simulink model "RST4"  (R2018a)
settings: Solver=VariableStepAuto  StartTime=0.0  StopTime=50  RelTol=1e-3
values from neighbouring files (symbols this model uses):
  A = den    [cod_teste_RST_4.m]
  B = num    [cod_teste_RST_4.m]
  ep = 0.9    [cod_teste_RST_4.m]
  p3 = Ap3(2)    [cod_teste_RST_4.m]
  p4 = Ap4(2)    [cod_teste_RST_4.m]
  R = [X(5) X(6) X(7) X(8)]    [cod_teste_RST_4.m]
  S = [X(1) X(2) X(3) X(4)]    [cod_teste_RST_4.m]
  T = sum(Am)/sum(B)    [cod_teste_RST_4.m]
  Ta = 0.1    [cod_teste_RST_4.m]
  tc = 1    [cod_teste_RST_4.m]
  Ts = 1    [cod_teste_RST_4.m]
libraries: dspinverses x1
settings Model: Creator=tarci  LastModifiedBy=tarci

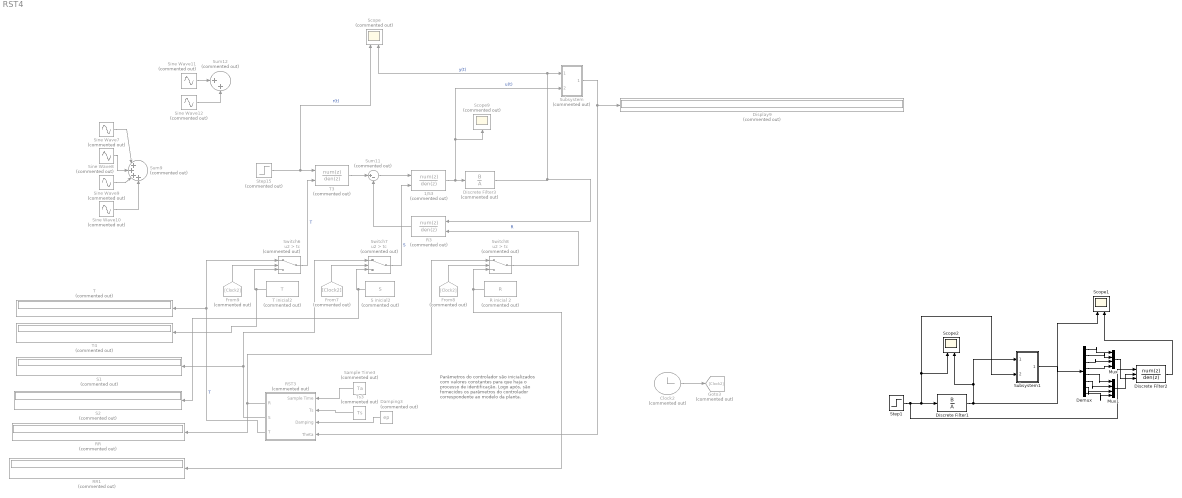
== system RST4 ==
  note: Parâmetros do controlador são inicializados
      | com valores constantes para que haja o
      | processo de identificação. Logo após, são
      | fornecidos os parâmetros do controlador
      | correspondente ao modelo da planta.
  1/S3 : DiscreteFilter  Commented=on  Numerator=1  DenominatorSource=Input port  Denominator=1  a0EqualsOne=on
      settings: InputPortMap=u0,p3
  Clock2 : Clock  Commented=on
  Damping3 : Constant  Commented=on  Value=ep
  Demux : Demux  Outputs=8
  Discrete Filter1 : DiscreteFilter  Numerator=B  Denominator=A  a0EqualsOne=on
  Discrete Filter2 : DiscreteFilter  NumeratorSource=Input port  Numerator=B  DenominatorSource=Input port  Denominator=A  a0EqualsOne=on
      settings: InputPortMap=u0,p1,p3
  Discrete Filter3 : DiscreteFilter  Commented=on  Numerator=B  Denominator=A  a0EqualsOne=on
  Display9 : Display  Commented=on
  From7 : From  Commented=on  GotoTag=Clock2
  From8 : From  Commented=on  GotoTag=Clock2
  From9 : From  Commented=on  GotoTag=Clock2
  Goto3 : Goto  Commented=on  GotoTag=Clock2
  Mux : Mux
  Mux1 : Mux
  R inicial 2 : Constant  Commented=on  Value=R
  R3 : DiscreteFilter  Commented=on  NumeratorSource=Input port  Numerator=[-620.2 131.3]  Denominator=1
      settings: InputPortMap=u0,p1
  RR : Display  Commented=on
  RR1 : Display  Commented=on
  RST3 : Subsystem  Commented=on
  S inicial2 : Constant  Commented=on  Value=S
  S1 : Display  Commented=on
  S2 : Display  Commented=on
  Sample Time3 : Constant  Commented=on  Value=Ta
  Scope : Scope  Commented=on  NumInputPorts=2
  Scope1 : Scope  NumInputPorts=2
  Scope2 : Scope  NumInputPorts=2
  Scope9 : Scope  Commented=on
  Sine Wave10 : Sin  Commented=on  Frequency=8  SampleTime=0
  Sine Wave11 : Sin  Commented=on  SampleTime=0
  Sine Wave12 : Sin  Commented=on  Frequency=2  SampleTime=0
  Sine Wave7 : Sin  Commented=on  SampleTime=0
  Sine Wave8 : Sin  Commented=on  Frequency=2  SampleTime=0
  Sine Wave9 : Sin  Commented=on  Frequency=4  SampleTime=0
  Step1 : Step  Time=0  SampleTime=0
  Step15 : Step  Commented=on  Time=0  SampleTime=0
  Subsystem : Subsystem  Commented=on
  Subsystem1 : Subsystem
  Sum11 : Sum  Commented=on  Inputs=|+-
  Sum12 : Sum  Commented=on  Inputs=|++
  Sum9 : Sum  Commented=on  Inputs=|++++
  Switch6 : Switch  Commented=on  Criteria=u2 > Threshold  Threshold=tc
  Switch7 : Switch  Commented=on  Criteria=u2 > Threshold  Threshold=tc
  Switch8 : Switch  Commented=on  Criteria=u2 > Threshold  Threshold=tc
  T : Display  Commented=on
  T inicial2 : Constant  Commented=on  Value=T
  T3 : DiscreteFilter  Commented=on  NumeratorSource=Input port  Numerator=13.39  Denominator=1
      settings: InputPortMap=u0,p1
  T4 : Display  Commented=on
  Ts3 : Constant  Commented=on  Value=Ts
  wires:
  Step15/1 -> Scope/1, T3/1  "r(t)"
  Sine Wave11/1 -> Sum12/1
  Discrete Filter3/1 -> R3/1, Subsystem/1(y(t)), Scope/2  "y(t)"
  Switch8/1 -> R3/2  "R"
  Sine Wave7/1 -> Sum9/1
  Sine Wave9/1 -> Sum9/3
  From9/1 -> Switch6/2
  Sine Wave8/1 -> Sum9/2
  T inicial2/1 -> T4/1, Switch6/3
  From7/1 -> Switch7/2
  1/S3/1 -> Subsystem/2("u(t) "), Scope9/1, Discrete Filter3/1  "u(t)"
  Subsystem/1("Theta(t) ") -> RST3/4(Theta), Display9/1
  T3/1 -> Sum11/1
  R3/1 -> Sum11/2
  Switch7/1 -> 1/S3/2  "S"
  Clock2/1 -> Goto3/1
  R inicial 2/1 -> RR1/1, Switch8/3
  Sum11/1 -> 1/S3/1
  Sine Wave12/1 -> Sum12/2
  Ts3/1 -> RST3/2(Ts)
  From8/1 -> Switch8/2
  Damping3/1 -> RST3/3(Damping)
  Sample Time3/1 -> RST3/1(Sample Time)
  RST3/3(T) -> Switch6/1, T/1  "T"
  RST3/1(R) -> Switch8/1, RR/1
  Sine Wave10/1 -> Sum9/4
  RST3/2(S) -> Switch7/1, S1/1
  S inicial2/1 -> S2/1, Switch7/3
  Switch6/1 -> T3/2  "T"
  Discrete Filter1/1 -> Scope1/1, Subsystem1/1(y(t)), Scope2/2
  Step1/1 -> Discrete Filter2/1, Subsystem1/2("u(t) "), Scope2/1, Discrete Filter1/1
  Subsystem1/1("Theta(t) ") -> Demux/1
  Demux/1 -> Mux/1
  Demux/2 -> Mux/2
  Demux/3 -> Mux/3
  Demux/4 -> Mux/4
  Demux/5 -> Mux1/1
  Demux/6 -> Mux1/2
  Demux/7 -> Mux1/3
  Demux/8 -> Mux1/4
  Mux1/1 -> Discrete Filter2/2
  Mux/1 -> Discrete Filter2/3
  Discrete Filter2/1 -> Scope1/2

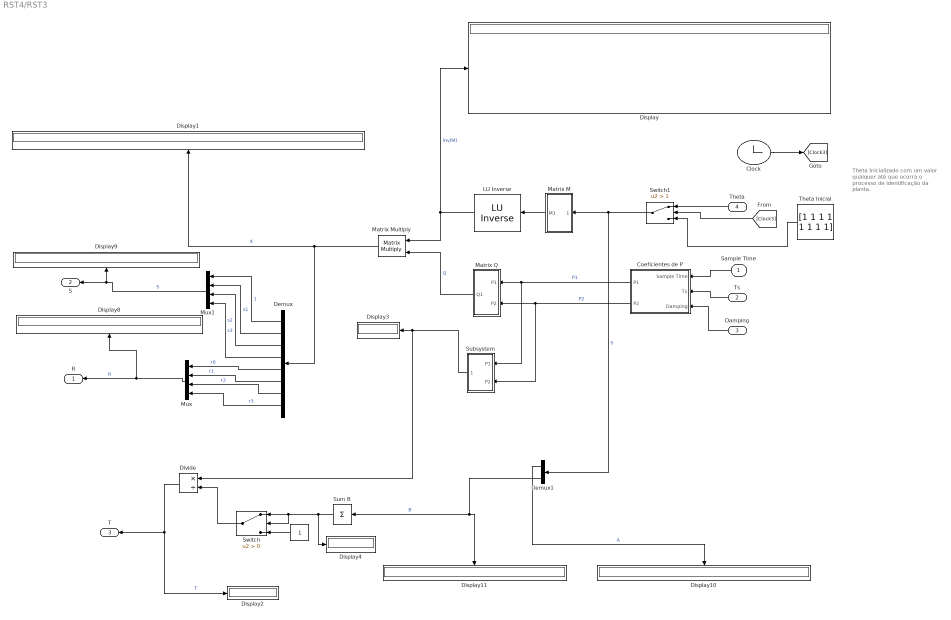
== system RST4/RST3 ==
  note: Theta Inicializado com um
      | valor qualquer até que ocorra
      |  o processo de identificação
      | da planta.
  Sample Time : Inport
  Ts : Inport  Port=2
  Damping : Inport  Port=3
  Theta : Inport  Port=4
  " " : Constant
  " LU Inverse" : dspinverses/ LU Inverse
      settings: SourceProductName=DSP System Toolbox
  Clock : Clock
  Coeficientes de P : Subsystem
  Demux : Demux  Outputs=8
  Demux1 : Demux  Outputs=2
  Display{,1..4,8..11} (9 alike) : Display
  Divide : Product  Inputs=*/
  Matrix M : Subsystem
  Matrix Multiply : Product  Multiplication=Matrix(*)
  Matrix Q : Subsystem
  Mux : Mux
  Mux1 : Mux
  Subsystem : Subsystem
  Sum B : Sum  Inputs=+
  Switch : Switch  Criteria=u2 > Threshold
  Switch1 : Switch  Criteria=u2 > Threshold  Threshold=1
  Theta Inicial : Constant  Value=[1 1 1 1 1 1 1 1]
  R : Outport
  S : Outport  Port=2
  T : Outport  Port=3
  wires:
  Matrix Multiply/1 -> Demux/1, Display1/1  "X"
  Sum B/1 -> Switch/2, Switch/1, Display4/1
  " LU Inverse"/1 -> Matrix Multiply/1, Display/1  "inv(M)"
  Mux1/1 -> S/1, Display9/1  "S"
  Coeficientes de P/2(P2) -> Subsystem/2(P2), Matrix Q/2(P2)  "P2"
  Divide/1 -> T/1, Display2/1  "T"
  Ts/1 -> Coeficientes de P/2(Ts)
  Damping/1 -> Coeficientes de P/3(Damping)
  Sample Time/1 -> Coeficientes de P/1(Sample Time)
  Coeficientes de P/1(P1) -> Subsystem/1(P1), Matrix Q/1(P1)  "P1"
  Demux1/2 -> Sum B/1, Display11/1  "B"
  Demux1/1 -> Display10/1  "A"
  Switch/1 -> Divide/2
  " "/1 -> Switch/3
  Mux/1 -> R/1, Display8/1  "R"
  Clock/1 -> [Clock3]
  Switch1/1 -> Matrix M/1(In1), Demux1/1  "S"
  Theta/1 -> Switch1/1
  [Clock3] -> Switch1/2
  Theta Inicial/1 -> Switch1/3
  Matrix Q/1(Q1) -> Matrix Multiply/2  "Q"
  Demux/1 -> Mux1/1  "1"
  Demux/2 -> Mux1/2  "s1"
  Matrix M/1(M1) -> " LU Inverse"/1
  Demux/3 -> Mux1/3  "s2"
  Demux/4 -> Mux1/4  "s3"
  Demux/5 -> Mux/1  "r0"
  Demux/6 -> Mux/2  "r1"
  Demux/7 -> Mux/3  "r2"
  Demux/8 -> Mux/4  "r3"
  Subsystem/1(Out1) -> Divide/1, Display3/1

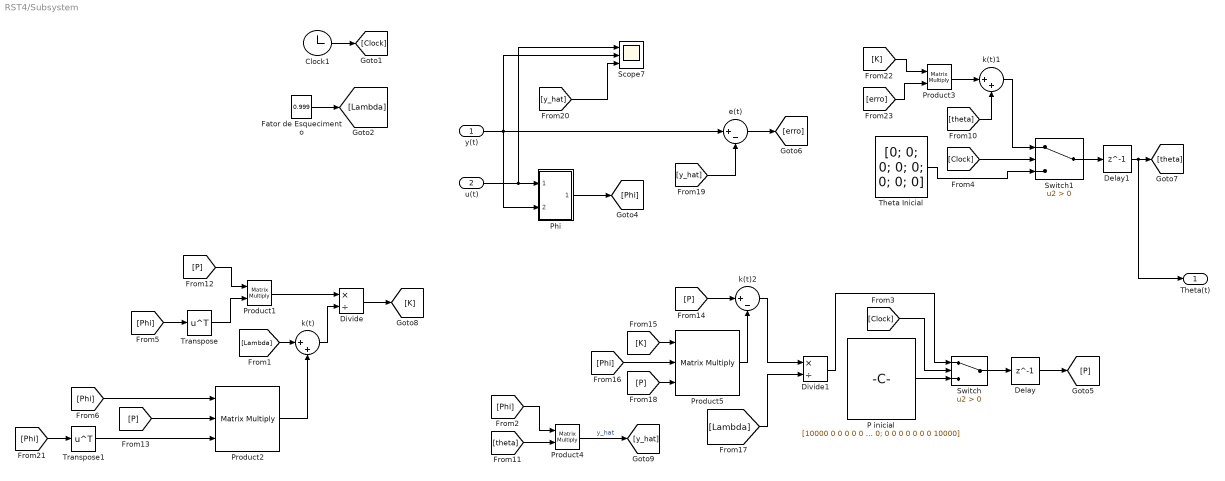
== system RST4/Subsystem ==
  y(t) : Inport
  "u(t) " : Inport  Port=2
  Clock1 : Clock
  Delay : Delay  DelayLength=1  InitialCondition=0
  Delay1 : Delay  DelayLength=1  InitialCondition=0
  Divide : Product  Inputs=*/
  Divide1 : Product  Inputs=*/
  "Fator de Esquecimento " : Constant  Value=0.999
  P inicial : Constant  Value=[10000 0 0 0 0 0 0 0; 0 10000 0 0 0 0 0 0; 0 0 10000 0 0 0 0 0; 0 0 0 10000 0 0 0 0; 0 0 0 0 10000 0 0 0; 0 0 0 0 0 10000 0 0; 0 0 0 0 0 0 10000 0; 0 0 0 0 0 0 0 10000]
  Phi : Subsystem
  Product1 : Product  Multiplication=Matrix(*)
  Product2 : Product  Inputs=3  Multiplication=Matrix(*)
  Product3 : Product  Multiplication=Matrix(*)
  Product4 : Product  Multiplication=Matrix(*)
  Product5 : Product  Inputs=3  Multiplication=Matrix(*)
  Scope7 : Scope  NumInputPorts=3
  Switch : Switch  Criteria=u2 > Threshold
  Switch1 : Switch  Criteria=u2 > Threshold
  "Theta Inicial " : Constant  Value=[0; 0; 0; 0; 0; 0; 0; 0]
  Transpose : Math  Operator=transpose  SaturateOnIntegerOverflow=on
  Transpose1 : Math  Operator=transpose  SaturateOnIntegerOverflow=on
  e(t) : Sum  Inputs=|+-
  k(t) : Sum  Inputs=|++
  k(t)1 : Sum  Inputs=|++
  k(t)2 : Sum  Inputs=|+-
  "Theta(t) " : Outport
  wires:
  k(t)/1 -> Divide/2
  [Phi] -> Product4/1
  Phi/1(Phi) -> [Phi]
  k(t)1/1 -> Switch1/1
  [y_hat] -> Scope7/3
  Switch1/1 -> Delay1/1
  [K] -> Product3/1
  Product2/1 -> k(t)/2
  [Clock] -> Switch1/2
  y(t)/1 -> e(t)/1, Scope7/2, Phi/2(y(t))
  k(t)2/1 -> Divide1/1
  Delay1/1 -> "Theta(t) "/1, [theta]
  Product5/1 -> k(t)2/2
  "u(t) "/1 -> Scope7/1, Phi/1(u(t))
  Switch/1 -> Delay/1
  [Lambda] -> Divide1/2
  Product1/1 -> Divide/1
  e(t)/1 -> [erro]
  Product3/1 -> k(t)1/1
  Delay/1 -> [P]
  [Phi] -> Transpose1/1
  [P] -> Product5/3
  "Fator de Esquecimento "/1 -> [Lambda]
  "Theta Inicial "/1 -> Switch1/3
  Transpose1/1 -> Product2/3
  Divide1/1 -> Switch/1
  [Phi] -> Transpose/1
  [Clock] -> Switch/2
  [theta] -> Product4/2
  [P] -> k(t)2/1
  [theta] -> k(t)1/2
  [P] -> Product2/2
  [Lambda] -> k(t)/1
  Transpose/1 -> Product1/2
  Clock1/1 -> [Clock]
  [erro] -> Product3/2
  [y_hat] -> e(t)/2
  [K] -> Product5/1
  P inicial/1 -> Switch/3
  [P] -> Product1/1
  [Phi] -> Product2/1
  Divide/1 -> [K]
  [Phi] -> Product5/2
  Product4/1 -> [y_hat]  "y_hat"

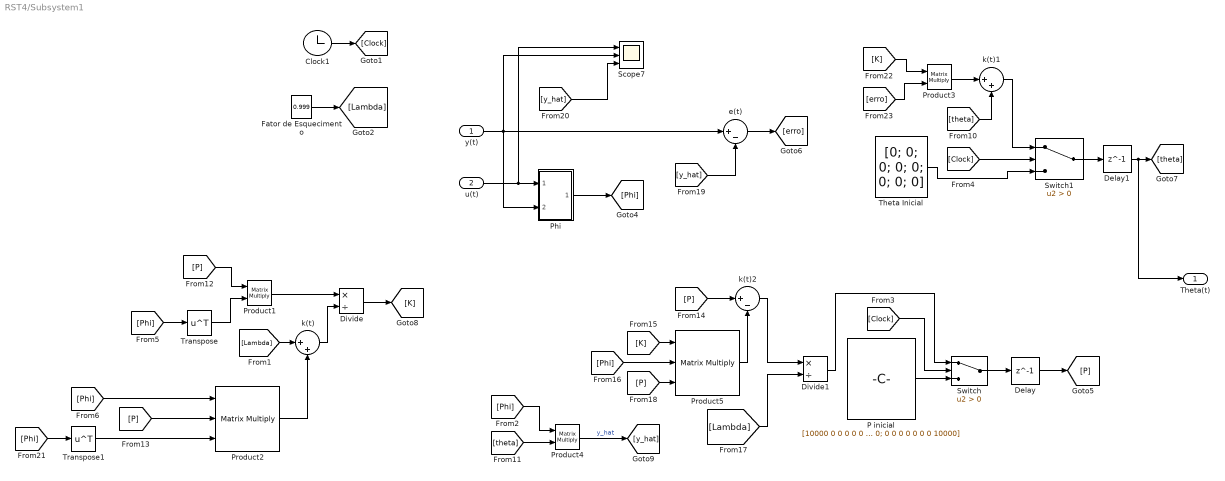
== system RST4/Subsystem1 ==
  y(t) : Inport
  "u(t) " : Inport  Port=2
  Clock1 : Clock
  Delay : Delay  DelayLength=1  InitialCondition=0
  Delay1 : Delay  DelayLength=1  InitialCondition=0
  Divide : Product  Inputs=*/
  Divide1 : Product  Inputs=*/
  "Fator de Esquecimento " : Constant  Value=0.999
  P inicial : Constant  Value=[10000 0 0 0 0 0 0 0; 0 10000 0 0 0 0 0 0; 0 0 10000 0 0 0 0 0; 0 0 0 10000 0 0 0 0; 0 0 0 0 10000 0 0 0; 0 0 0 0 0 10000 0 0; 0 0 0 0 0 0 10000 0; 0 0 0 0 0 0 0 10000]
  Phi : Subsystem
  Product1 : Product  Multiplication=Matrix(*)
  Product2 : Product  Inputs=3  Multiplication=Matrix(*)
  Product3 : Product  Multiplication=Matrix(*)
  Product4 : Product  Multiplication=Matrix(*)
  Product5 : Product  Inputs=3  Multiplication=Matrix(*)
  Scope7 : Scope  NumInputPorts=3
  Switch : Switch  Criteria=u2 > Threshold
  Switch1 : Switch  Criteria=u2 > Threshold
  "Theta Inicial " : Constant  Value=[0; 0; 0; 0; 0; 0; 0; 0]
  Transpose : Math  Operator=transpose  SaturateOnIntegerOverflow=on
  Transpose1 : Math  Operator=transpose  SaturateOnIntegerOverflow=on
  e(t) : Sum  Inputs=|+-
  k(t) : Sum  Inputs=|++
  k(t)1 : Sum  Inputs=|++
  k(t)2 : Sum  Inputs=|+-
  "Theta(t) " : Outport
  wires:
  Product4/1 -> [y_hat]  "y_hat"
  [Phi] -> Product5/2
  Divide/1 -> [K]
  [Phi] -> Product2/1
  [P] -> Product1/1
  P inicial/1 -> Switch/3
  [K] -> Product5/1
  [y_hat] -> e(t)/2
  [erro] -> Product3/2
  Clock1/1 -> [Clock]
  Transpose/1 -> Product1/2
  [Lambda] -> k(t)/1
  [P] -> Product2/2
  [theta] -> k(t)1/2
  [P] -> k(t)2/1
  [theta] -> Product4/2
  [Clock] -> Switch/2
  [Phi] -> Transpose/1
  Divide1/1 -> Switch/1
  Transpose1/1 -> Product2/3
  "Theta Inicial "/1 -> Switch1/3
  "Fator de Esquecimento "/1 -> [Lambda]
  [P] -> Product5/3
  [Phi] -> Transpose1/1
  Delay/1 -> [P]
  Product3/1 -> k(t)1/1
  e(t)/1 -> [erro]
  Product1/1 -> Divide/1
  [Lambda] -> Divide1/2
  Switch/1 -> Delay/1
  "u(t) "/1 -> Phi/1(u(t)), Scope7/1
  Product5/1 -> k(t)2/2
  Delay1/1 -> [theta], "Theta(t) "/1
  k(t)2/1 -> Divide1/1
  y(t)/1 -> Phi/2(y(t)), Scope7/2, e(t)/1
  [Clock] -> Switch1/2
  Product2/1 -> k(t)/2
  [K] -> Product3/1
  Switch1/1 -> Delay1/1
  [y_hat] -> Scope7/3
  k(t)1/1 -> Switch1/1
  Phi/1(Phi) -> [Phi]
  [Phi] -> Product4/1
  k(t)/1 -> Divide/2

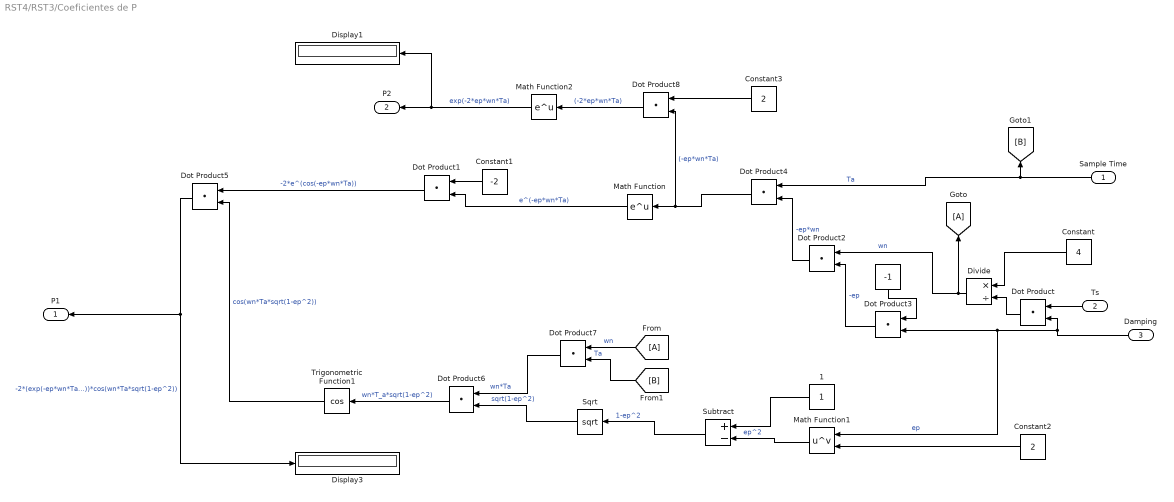
== system RST4/RST3/Coeficientes de P ==
  Sample Time : Inport
  Ts : Inport  Port=2
  Damping : Inport  Port=3
  " " : Constant  Value=-1
  1 : Constant
  Constant : Constant  Value=4
  Constant1 : Constant  Value=-2
  Constant2 : Constant  Value=2
  Constant3 : Constant  Value=2
  Display1 : Display
  Display3 : Display
  Divide : Product  Inputs=*/
  Dot Product{,1..8} (9 alike) : DotProduct  InputSameDT=on  OutDataTypeStr=Inherit: Inherit via internal rule
  Math Function : Math  SaturateOnIntegerOverflow=on
  Math Function1 : Math  Operator=pow  SaturateOnIntegerOverflow=on
  Math Function2 : Math  SaturateOnIntegerOverflow=on
  Sqrt : Sqrt  SaturateOnIntegerOverflow=on
  Subtract : Sum  Inputs=+-
  Trigonometric Function1 : Trigonometry  Operator=cos
  P1 : Outport
  P2 : Outport  Port=2
  wires:
  Math Function/1 -> Dot Product1/2  "e^(-ep*wn*Ta)"
  Divide/1 -> [A], Dot Product2/1  "wn"
  [A] -> Dot Product7/1  "wn"
  " "/1 -> Dot Product3/1
  Dot Product5/1 -> P1/1, Display3/1  "-2*(exp(-ep*wn*Ta))*cos(wn*Ta*sqrt(1-ep^2))"
  Trigonometric Function1/1 -> Dot Product5/2  "cos(wn*Ta*sqrt(1-ep^2))"
  Ts/1 -> Dot Product/1
  Dot Product/1 -> Divide/2
  Dot Product3/1 -> Dot Product2/2  "-ep"
  Damping/1 -> Math Function1/1, Dot Product3/2, Dot Product/2  "ep"
  Constant/1 -> Divide/1
  Dot Product7/1 -> Dot Product6/1  "wn*Ta"
  Sample Time/1 -> Dot Product4/1, [B]  "Ta"
  Math Function1/1 -> Subtract/2  "ep^2"
  Dot Product1/1 -> Dot Product5/1  "-2*e^(cos(-ep*wn*Ta))"
  Constant2/1 -> Math Function1/2
  1/1 -> Subtract/1
  Constant1/1 -> Dot Product1/1
  Dot Product2/1 -> Dot Product4/2  "-ep*wn"
  [B] -> Dot Product7/2  "Ta"
  Dot Product6/1 -> Trigonometric Function1/1  "wn*T_a*sqrt(1-ep^2)"
  Dot Product4/1 -> Dot Product8/2, Math Function/1  "(-ep*wn*Ta)"
  Sqrt/1 -> Dot Product6/2  "sqrt(1-ep^2)"
  Subtract/1 -> Sqrt/1  "1-ep^2"
  Constant3/1 -> Dot Product8/1
  Dot Product8/1 -> Math Function2/1  "(-2*ep*wn*Ta)"
  Math Function2/1 -> Display1/1, P2/1  "exp(-2*ep*wn*Ta)"

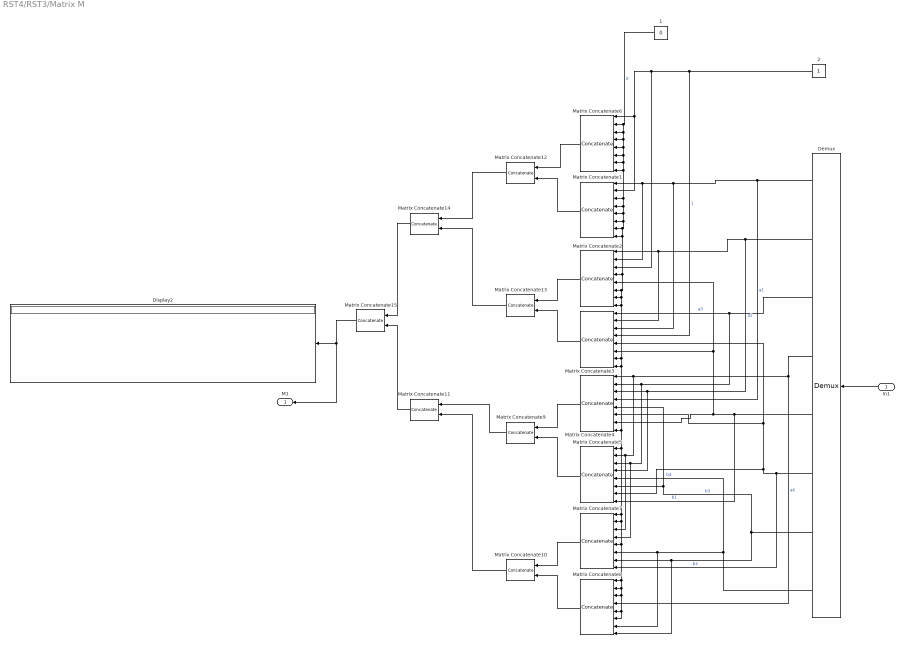
== system RST4/RST3/Matrix M ==
  In1 : Inport
  " 1" : Constant  Value=0
  2 : Constant
  Demux : Demux  Outputs=8
  Display2 : Display
  Matrix Concatenate{1..8} (8 alike) : Concatenate  NumInputs=8  Mode=Multidimensional array  ConcatenateDimension=2
  Matrix Concatenate{9..15} (7 alike) : Concatenate  Mode=Multidimensional array
  M1 : Outport
  wires:
  In1/1 -> Demux/1
  2/1 -> Matrix Concatenate3/4, Matrix Concatenate2/3, Matrix Concatenate1/2, Matrix Concatenate6/1  "1"
  Matrix Concatenate6/1 -> Matrix Concatenate12/1
  Matrix Concatenate13/1 -> Matrix Concatenate14/2
  Matrix Concatenate12/1 -> Matrix Concatenate14/1
  Matrix Concatenate9/1 -> Matrix Concatenate11/1
  Matrix Concatenate10/1 -> Matrix Concatenate11/2
  Matrix Concatenate14/1 -> Matrix Concatenate15/1
  Matrix Concatenate11/1 -> Matrix Concatenate15/2
  Matrix Concatenate15/1 -> M1/1, Display2/1
  Matrix Concatenate1/1 -> Matrix Concatenate12/2
  Matrix Concatenate2/1 -> Matrix Concatenate13/1
  Matrix Concatenate3/1 -> Matrix Concatenate13/2
  Matrix Concatenate4/1 -> Matrix Concatenate9/1
  Matrix Concatenate5/1 -> Matrix Concatenate9/2
  Matrix Concatenate7/1 -> Matrix Concatenate10/1
  Matrix Concatenate8/1 -> Matrix Concatenate10/2
  " 1"/1 -> Matrix Concatenate8/6, Matrix Concatenate8/5, Matrix Concatenate8/3, Matrix Concatenate8/2, Matrix Concatenate8/1, Matrix Concatenate7/5, Matrix Concatenate7/2, Matrix Concatenate7/1, Matrix Concatenate5/1, Matrix Concatenate4/8, Matrix Concatenate3/8, Matrix Concatenate3/7, Matrix Concatenate2/8, Matrix Concatenate2/7, Matrix Concatenate2/6, Matrix Concatenate2/4, Matrix Concatenate1/8, Matrix Concatenate1/7, Matrix Concatenate1/6, Matrix Concatenate1/5, Matrix Concatenate1/4, Matrix Concatenate1/3, Matrix Concatenate6/8, Matrix Concatenate6/7, Matrix Concatenate6/6, Matrix Concatenate6/5, Matrix Concatenate6/4, Matrix Concatenate6/3, Matrix Concatenate6/2  "0"
  Demux/1 -> Matrix Concatenate4/4, Matrix Concatenate3/3, Matrix Concatenate2/2, Matrix Concatenate1/1  "a1"
  Demux/2 -> Matrix Concatenate5/4, Matrix Concatenate4/3, Matrix Concatenate3/2, Matrix Concatenate2/1  "a2"
  Demux/5 -> Matrix Concatenate5/8, Matrix Concatenate4/7, Matrix Concatenate3/6, Matrix Concatenate2/5  "b1"
  Demux/3 -> Matrix Concatenate7/4, Matrix Concatenate5/3, Matrix Concatenate4/2, Matrix Concatenate3/1  "a3"
  Demux/6 -> Matrix Concatenate7/8, Matrix Concatenate5/7, Matrix Concatenate4/6, Matrix Concatenate3/5  "b2"
  Demux/4 -> Matrix Concatenate8/4, Matrix Concatenate7/3, Matrix Concatenate5/2, Matrix Concatenate4/1  "a4"
  Demux/7 -> Matrix Concatenate5/6, Matrix Concatenate4/5, Matrix Concatenate8/8, Matrix Concatenate7/7  "b3"
  Demux/8 -> Matrix Concatenate8/7, Matrix Concatenate7/6, Matrix Concatenate5/5  "b4"

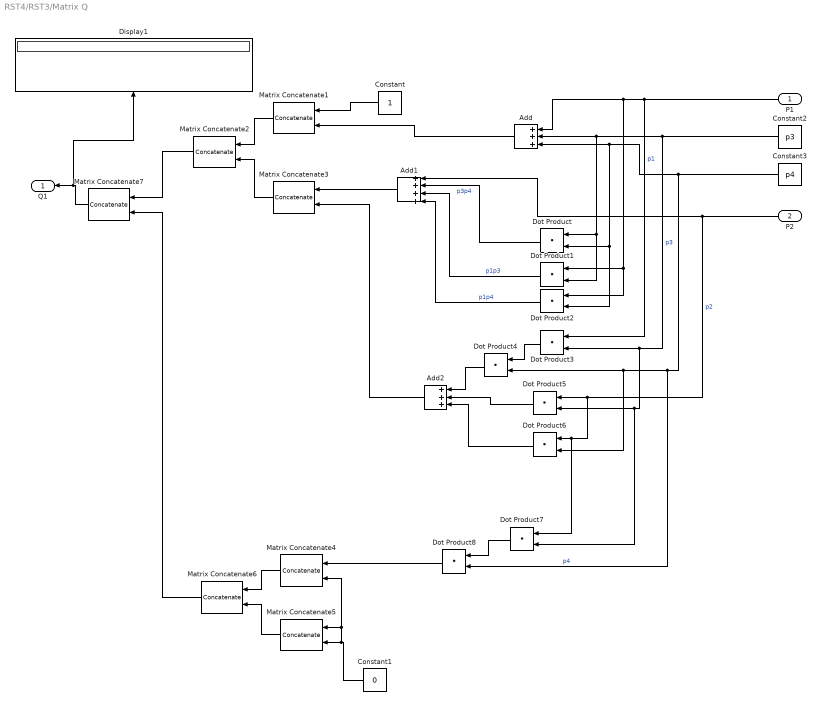
== system RST4/RST3/Matrix Q ==
  P1 : Inport
  P2 : Inport  Port=2
  Add : Sum  Inputs=+++
  Add1 : Sum  Inputs=++++
  Add2 : Sum  Inputs=+++
  Constant : Constant
  Constant1 : Constant  Value=0
  Constant2 : Constant  Value=p3
  Constant3 : Constant  Value=p4
  Display1 : Display
  Dot Product{,1..8} (9 alike) : DotProduct  InputSameDT=on  OutDataTypeStr=Inherit: Inherit via internal rule
  Matrix Concatenate{1..7} (7 alike) : Concatenate  Mode=Multidimensional array
  Q1 : Outport
  wires:
  Matrix Concatenate1/1 -> Matrix Concatenate2/1
  Matrix Concatenate3/1 -> Matrix Concatenate2/2
  Constant/1 -> Matrix Concatenate1/1
  P1/1 -> Dot Product3/1, Dot Product2/1, Dot Product1/1, Add/1  "p1"
  Add/1 -> Matrix Concatenate1/2
  Constant2/1 -> Dot Product7/2, Dot Product5/2, Dot Product3/2, Dot Product1/2, Dot Product/1, Add/2  "p3"
  Constant3/1 -> Dot Product8/2, Dot Product6/2, Dot Product4/2, Dot Product2/2, Dot Product/2, Add/3  "p4"
  P2/1 -> Dot Product7/1, Dot Product6/1, Dot Product5/1, Add1/1  "p2"
  Dot Product/1 -> Add1/2  "p3p4"
  Dot Product1/1 -> Add1/3  "p1p3"
  Dot Product2/1 -> Add1/4  "p1p4"
  Add1/1 -> Matrix Concatenate3/1
  Matrix Concatenate7/1 -> Display1/1, Q1/1
  Matrix Concatenate2/1 -> Matrix Concatenate7/1
  Matrix Concatenate4/1 -> Matrix Concatenate6/1
  Matrix Concatenate5/1 -> Matrix Concatenate6/2
  Matrix Concatenate6/1 -> Matrix Concatenate7/2
  Dot Product3/1 -> Dot Product4/1
  Dot Product5/1 -> Add2/2
  Dot Product6/1 -> Add2/3
  Dot Product4/1 -> Add2/1
  Add2/1 -> Matrix Concatenate3/2
  Constant1/1 -> Matrix Concatenate4/2, Matrix Concatenate5/1, Matrix Concatenate5/2
  Dot Product7/1 -> Dot Product8/1
  Dot Product8/1 -> Matrix Concatenate4/1

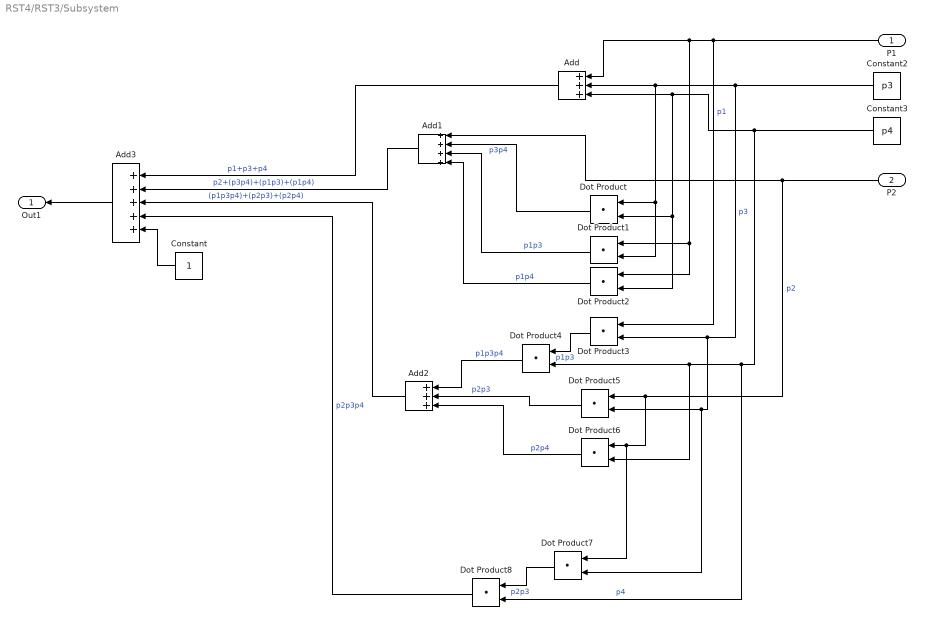
== system RST4/RST3/Subsystem ==
  P1 : Inport
  P2 : Inport  Port=2
  Add : Sum  Inputs=+++
  Add1 : Sum  Inputs=++++
  Add2 : Sum  Inputs=+++
  Add3 : Sum  Inputs=+++++
  Constant : Constant
  Constant2 : Constant  Value=p3
  Constant3 : Constant  Value=p4
  Dot Product{,1..8} (9 alike) : DotProduct  InputSameDT=on  OutDataTypeStr=Inherit: Inherit via internal rule
  Out1 : Outport
  wires:
  Add1/1 -> Add3/2  "p2+(p3p4)+(p1p3)+(p1p4)"
  Add/1 -> Add3/1  "p1+p3+p4"
  Add3/1 -> Out1/1
  Constant2/1 -> Dot Product7/2, Dot Product5/2, Dot Product3/2, Dot Product1/2, Dot Product/1, Add/2  "p3"
  Constant3/1 -> Dot Product8/2, Dot Product6/2, Dot Product4/2, Dot Product2/2, Dot Product/2, Add/3  "p4"
  P2/1 -> Dot Product7/1, Dot Product6/1, Dot Product5/1, Add1/1  "p2"
  P1/1 -> Dot Product3/1, Dot Product2/1, Dot Product1/1, Add/1  "p1"
  Dot Product1/1 -> Add1/3  "p1p3"
  Dot Product2/1 -> Add1/4  "p1p4"
  Dot Product6/1 -> Add2/3  "p2p4"
  Dot Product5/1 -> Add2/2  "p2p3"
  Dot Product4/1 -> Add2/1  "p1p3p4"
  Add2/1 -> Add3/3  "(p1p3p4)+(p2p3)+(p2p4)"
  Dot Product8/1 -> Add3/4  "p2p3p4"
  Dot Product/1 -> Add1/2  "p3p4"
  Dot Product3/1 -> Dot Product4/1  "p1p3"
  Dot Product7/1 -> Dot Product8/1  "p2p3"
  Constant/1 -> Add3/5

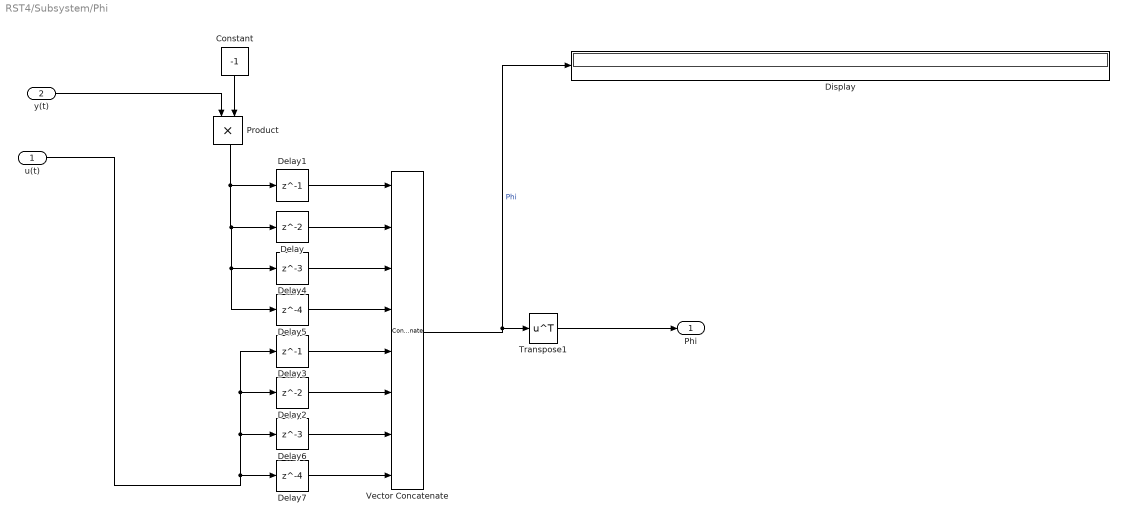
== system RST4/Subsystem/Phi ==
  u(t) : Inport
  y(t) : Inport  Port=2
  Constant : Constant  Value=-1
  Delay : Delay
  Delay1 : Delay  DelayLength=1
  Delay2 : Delay
  Delay3 : Delay  DelayLength=1
  Delay4 : Delay  DelayLength=3
  Delay5 : Delay  DelayLength=4
  Delay6 : Delay  DelayLength=3
  Delay7 : Delay  DelayLength=4
  Display : Display
  Product : Product
  Transpose1 : Math  Operator=transpose  SaturateOnIntegerOverflow=on
  Vector Concatenate : Concatenate  NumInputs=8
  Phi : Outport
  wires:
  Vector Concatenate/1 -> Display/1, Transpose1/1  "Phi"
  Delay/1 -> Vector Concatenate/2
  y(t)/1 -> Product/1
  Delay1/1 -> Vector Concatenate/1
  Transpose1/1 -> Phi/1
  Constant/1 -> Product/2
  Product/1 -> Delay5/1, Delay4/1, Delay/1, Delay1/1
  Delay4/1 -> Vector Concatenate/3
  Delay5/1 -> Vector Concatenate/4
  Delay3/1 -> Vector Concatenate/5
  Delay2/1 -> Vector Concatenate/6
  Delay6/1 -> Vector Concatenate/7
  Delay7/1 -> Vector Concatenate/8
  u(t)/1 -> Delay7/1, Delay6/1, Delay2/1, Delay3/1

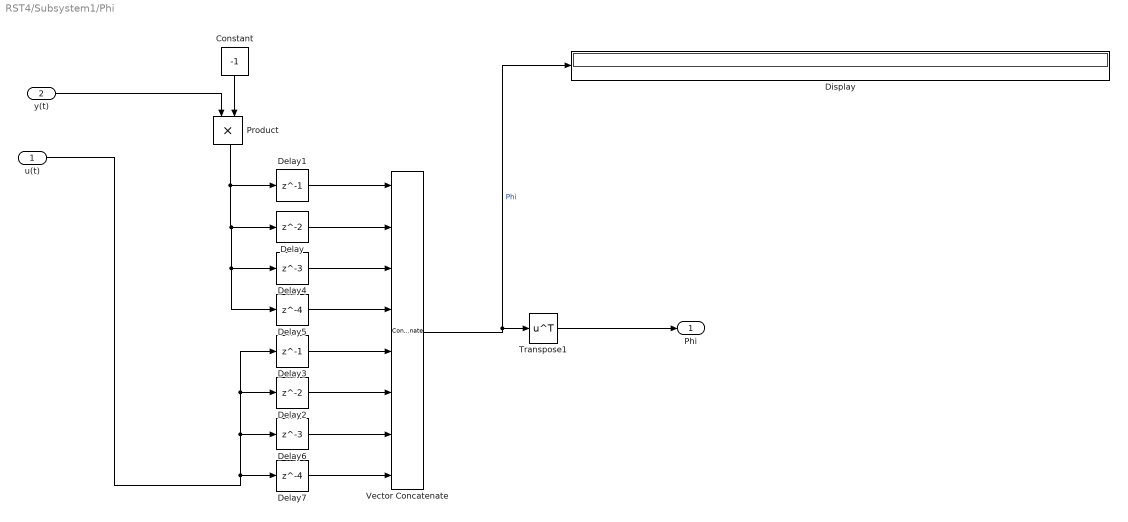
== system RST4/Subsystem1/Phi ==
  u(t) : Inport
  y(t) : Inport  Port=2
  Constant : Constant  Value=-1
  Delay : Delay
  Delay1 : Delay  DelayLength=1
  Delay2 : Delay
  Delay3 : Delay  DelayLength=1
  Delay4 : Delay  DelayLength=3
  Delay5 : Delay  DelayLength=4
  Delay6 : Delay  DelayLength=3
  Delay7 : Delay  DelayLength=4
  Display : Display
  Product : Product
  Transpose1 : Math  Operator=transpose  SaturateOnIntegerOverflow=on
  Vector Concatenate : Concatenate  NumInputs=8
  Phi : Outport
  wires:
  u(t)/1 -> Delay3/1, Delay2/1, Delay6/1, Delay7/1
  Delay7/1 -> Vector Concatenate/8
  Delay6/1 -> Vector Concatenate/7
  Delay2/1 -> Vector Concatenate/6
  Delay3/1 -> Vector Concatenate/5
  Delay5/1 -> Vector Concatenate/4
  Delay4/1 -> Vector Concatenate/3
  Product/1 -> Delay1/1, Delay/1, Delay4/1, Delay5/1
  Constant/1 -> Product/2
  Transpose1/1 -> Phi/1
  Delay1/1 -> Vector Concatenate/1
  y(t)/1 -> Product/1
  Delay/1 -> Vector Concatenate/2
  Vector Concatenate/1 -> Transpose1/1, Display/1  "Phi"
